simulink model "lotka_volterra"  (R2023a)
settings: Solver=ode15s  StartTime=0.0  StopTime=10.0  RelTol=1e-3
settings Model: Creator=Kami Valle  LastModifiedBy=Kami Valle
settings DataIOCC: ReturnWorkspaceOutputs=off  TimeSaveName=t

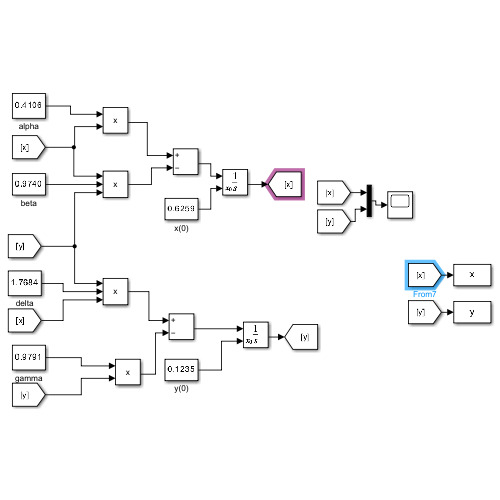
[thumbnail: Simulink's stored preview of the top-level diagram]
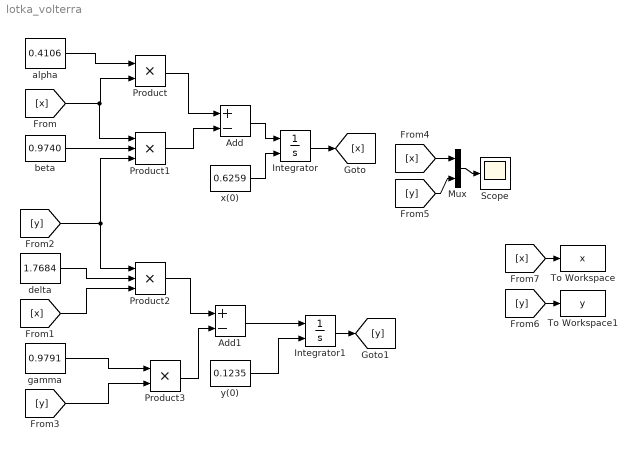
== system lotka_volterra ==
  Add : Sum  Inputs=+-
  Add1 : Sum  Inputs=+-
  Integrator : Integrator  InitialConditionSource=external
  Integrator1 : Integrator  InitialConditionSource=external
  Mux : Mux  Inputs=2
  Product : Product
  Product1 : Product  Inputs=3
  Product2 : Product  Inputs=3
  Product3 : Product
  Scope : Scope
  To Workspace : ToWorkspace  VariableName=x  SampleTime=-1
  To Workspace1 : ToWorkspace  VariableName=y  SampleTime=-1
  alpha : Constant  Value=0.4106
  beta : Constant  Value=0.9740
  delta : Constant  Value=1.7684
  gamma : Constant  Value=0.9791
  x(0) : Constant  Value=0.6259
  y(0) : Constant  Value=0.1235
  wires:
  alpha/1 -> Product/1
  Product/1 -> Add/1
  Product1/1 -> Add/2
  beta/1 -> Product1/2
  gamma/1 -> Product3/1
  Add/1 -> Integrator/1
  x(0)/1 -> Integrator/2
  Integrator/1 -> [x]
  [x] -> Product1/1, Product/2
  [x] -> Product2/3
  delta/1 -> Product2/2
  [y] -> Product3/2
  [y] -> Product1/3, Product2/1
  Product2/1 -> Add1/1
  Product3/1 -> Add1/2
  Add1/1 -> Integrator1/1
  y(0)/1 -> Integrator1/2
  Integrator1/1 -> [y]
  Mux/1 -> Scope/1
  [x] -> Mux/1
  [y] -> Mux/2
  [y] -> To Workspace1/1
  [x] -> To Workspace/1
